simulink model "HW4_final_"  (Simulink 7.9)
settings: Solver=ode45  StartTime=0.0  StopTime=200.0  RelTol=1e-3
settings Model: Creator=alex  LastModifiedBy=alex
settings CodeAppCC: CustomSymbolStrType=$N$R$M_T

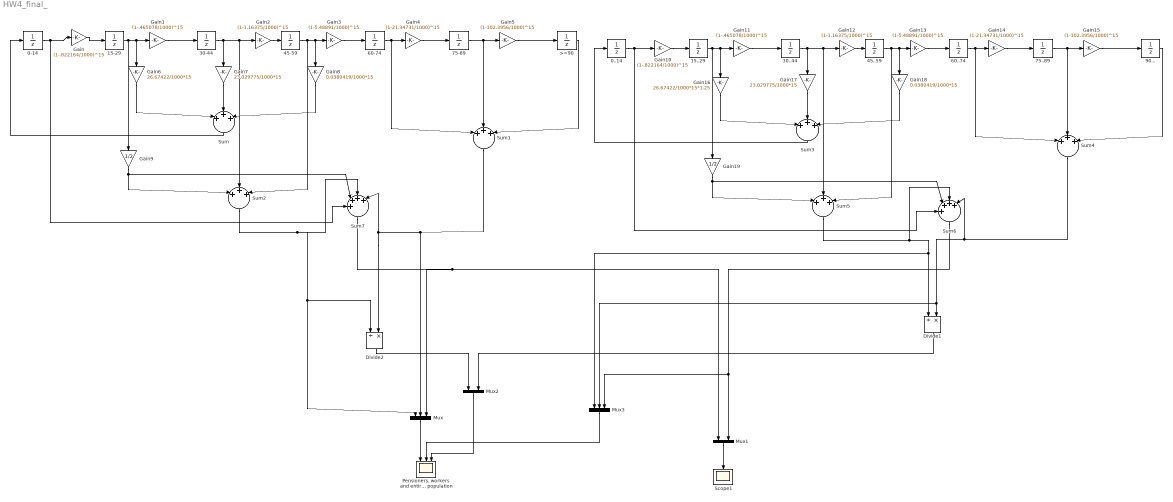
== system HW4_final_ ==
  0-14 : UnitDelay  X0=1494370  SampleTime=15
  0..14 : UnitDelay  X0=1494370  SampleTime=15
  15-29 : UnitDelay  X0=2075652  SampleTime=15
  15..29 : UnitDelay  X0=2075652  SampleTime=15
  30-44 : UnitDelay  X0=2474329  SampleTime=15
  30..44 : UnitDelay  X0=2474329  SampleTime=15
  45-59 : UnitDelay  X0=2142379  SampleTime=15
  45..59 : UnitDelay  X0=2142379  SampleTime=15
  60-74 : UnitDelay  X0=1626214  SampleTime=15
  60..74 : UnitDelay  X0=1626214  SampleTime=15
  75-89 : UnitDelay  X0=665283  SampleTime=15
  75..89 : UnitDelay  X0=665283  SampleTime=15
  90... : UnitDelay  X0=28586  SampleTime=15
  >=90 : UnitDelay  X0=28586  SampleTime=15
  Divide1 : Product  Inputs=/*
  Divide2 : Product  Inputs=/*
  Gain : Gain  Gain=(1-.822164/1000)^15
  Gain1 : Gain  Gain=(1-.465078/1000)^15
  Gain10 : Gain  Gain=(1-.822164/1000)^15
  Gain11 : Gain  Gain=(1-.465078/1000)^15
  Gain12 : Gain  Gain=(1-1.16375/1000)^15
  Gain13 : Gain  Gain=(1-5.48891/1000)^15
  Gain14 : Gain  Gain=(1-21.34731/1000)^15
  Gain15 : Gain  Gain=(1-102.3956/1000)^15
  Gain16 : Gain  Gain=26.67422/1000*15*1.25
  Gain17 : Gain  Gain=23.029775/1000*15
  Gain18 : Gain  Gain=0.0380419/1000*15
  Gain19 : Gain  Gain=1/2
  Gain2 : Gain  Gain=(1-1.16375/1000)^15
  Gain3 : Gain  Gain=(1-5.48891/1000)^15
  Gain4 : Gain  Gain=(1-21.34731/1000)^15
  Gain5 : Gain  Gain=(1-102.3956/1000)^15
  Gain6 : Gain  Gain=26.67422/1000*15
  Gain7 : Gain  Gain=23.029775/1000*15
  Gain8 : Gain  Gain=0.0380419/1000*15
  Gain9 : Gain  Gain=1/2
  Mux : Mux  Inputs=3
  Mux1 : Mux  Inputs=2
  Mux2 : Mux  Inputs=2
  Mux3 : Mux  Inputs=3
  "Pensioners, workers and entire population " : Scope  NumInputPorts=3
      settings: YMin=-5~-5~-5  YMax=5~5~5
  Scope1 : Scope
  Sum{,1..5} (6 alike) : Sum  Inputs=|+|+|+|
  Sum6 : Sum  Inputs=++++|
  Sum7 : Sum  Inputs=++++|
  wires:
  Sum/1 -> 0-14/1
  Gain6/1 -> Sum/1
  Gain7/1 -> Sum/2
  15-29/1 -> Gain1/1, Gain6/1, Gain9/1
  Gain1/1 -> 30-44/1
  30-44/1 -> Gain7/1, Gain2/1, Sum2/2
  Gain2/1 -> 45-59/1
  45-59/1 -> Gain3/1, Gain8/1, Sum2/3
  Gain3/1 -> 60-74/1
  60-74/1 -> Gain4/1, Sum1/1
  Gain4/1 -> 75-89/1
  75-89/1 -> Gain5/1, Sum1/2
  Gain5/1 -> >=90/1
  0-14/1 -> Sum7/1, Gain/1
  Gain/1 -> 15-29/1
  Gain8/1 -> Sum/3
  Gain9/1 -> Sum7/2, Sum2/1
  >=90/1 -> Sum1/3
  Sum2/1 -> Sum7/3, Mux/1, Divide2/1
  Sum1/1 -> Mux/2, Sum7/4, Divide2/2
  Sum3/1 -> 0..14/1
  Gain16/1 -> Sum3/1
  Gain17/1 -> Sum3/2
  15..29/1 -> Gain19/1, Gain11/1, Gain16/1
  Gain11/1 -> 30..44/1
  30..44/1 -> Sum5/2, Gain12/1, Gain17/1
  Gain12/1 -> 45..59/1
  45..59/1 -> Sum5/3, Gain18/1, Gain13/1
  Gain13/1 -> 60..74/1
  60..74/1 -> Sum4/1, Gain14/1
  Gain14/1 -> 75..89/1
  75..89/1 -> Sum4/2, Gain15/1
  Gain15/1 -> 90.../1
  0..14/1 -> Gain10/1, Sum6/1
  Gain10/1 -> 15..29/1
  Gain18/1 -> Sum3/3
  Gain19/1 -> Sum5/1, Sum6/2
  90.../1 -> Sum4/3
  Sum5/1 -> Sum6/3, Divide1/1, Mux3/1
  Sum4/1 -> Sum6/4, Divide1/2, Mux3/2
  Mux/1 -> "Pensioners, workers and entire population "/1
  Mux1/1 -> Scope1/1
  Sum7/1 -> Mux1/1, Mux/3
  Sum6/1 -> Mux1/2, Mux3/3
  Divide2/1 -> Mux2/1
  Divide1/1 -> Mux2/2
  Mux2/1 -> "Pensioners, workers and entire population "/3
  Mux3/1 -> "Pensioners, workers and entire population "/2
